simulink model "pyTrials"  (R2017a)
settings: Solver=VariableStepAuto  StartTime=0.0  StopTime=10.0  RelTol=1e-3
settings Model: Creator=Pablo Diaz  LastModifiedBy=Pablo Diaz

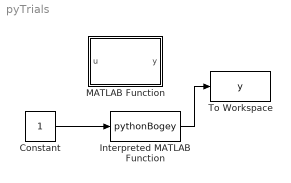
== system pyTrials ==
  Constant : Constant
  Interpreted MATLAB Function : MATLABFcn  MATLABFcn=pythonBogey
  MATLAB Function : MATLAB Function  TreatAsAtomicUnit=on
  To Workspace : ToWorkspace  VariableName=y  SaveFormat=Timeseries  SampleTime=-1
  wires:
  Constant/1 -> Interpreted MATLAB Function/1
  Interpreted MATLAB Function/1 -> To Workspace/1

== matlab function pyTrials/MATLAB Function ==
  data: u input; y output
function y = fcn(u)
% N = py.list({'Jones','Johnson','James'});
% names = py.mymod.search(N);
y = 100*u;
